simulink model "ACS_LON_AP_MODAL_INTEGRAL"  (R2022b)
settings: Solver=VariableStepAuto  StartTime=0.0  StopTime=inf  RelTol=1e-3
libraries: cstblocks x1
settings Model: Creator=bendr  LastModifiedBy=bendr

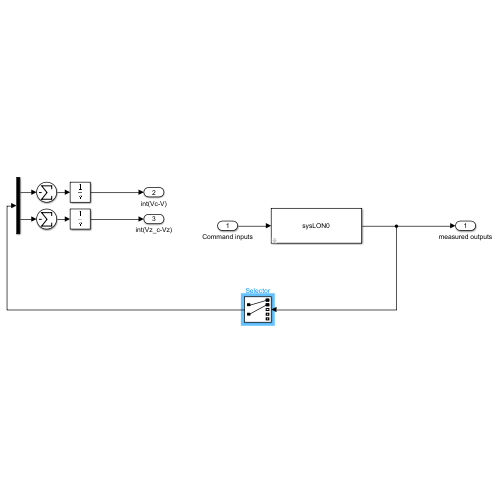
[thumbnail: Simulink's stored preview of the top-level diagram]
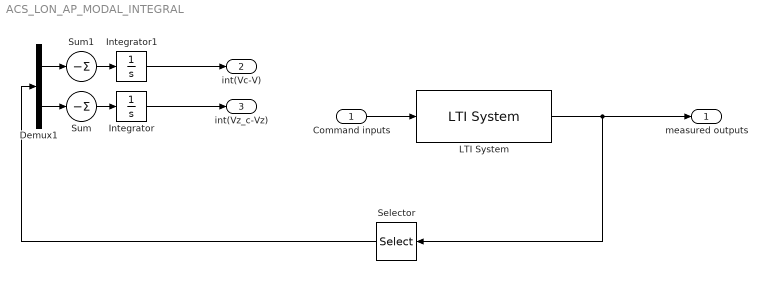
== system ACS_LON_AP_MODAL_INTEGRAL ==
  Command inputs : Inport
  Demux1 : Demux  Outputs=2
  Integrator : Integrator
  Integrator1 : Integrator
  LTI System : cstblocks/LTI System  sys=sysLON0  IC=[]
  Selector : Selector  InputPortWidth=5  IndexOptions=Index vector (dialog)  Indices=[1 2]  OutputSizes=1
  Sum : Sum  Inputs=-
  Sum1 : Sum  Inputs=-
  measured outputs : Outport
  int(Vc-V) : Outport  Port=2
  int(Vz_c-Vz) : Outport  Port=3
  wires:
  LTI System/1 -> Selector/1, measured outputs/1
  Command inputs/1 -> LTI System/1
  Integrator1/1 -> int(Vc-V)/1
  Integrator/1 -> int(Vz_c-Vz)/1
  Demux1/2 -> Sum/1
  Sum/1 -> Integrator/1
  Selector/1 -> Demux1/1
  Sum1/1 -> Integrator1/1
  Demux1/1 -> Sum1/1
